simulink library "frdc"  (Simulink 8.1)
settings: Solver=ode1  StartTime=0.0  StopTime=Inf  FixedStep=0.001  RelTol=1e-3
PostLoadFcn:
  | , if any(exist('dsrtsu_mdlpostloadfcn', 'file') == [2, 3, 6]), try dsrtsu_mdlpostloadfcn('Execute', bdroot); catch fprintf('Error in PostLoadFcn (dsrtsu_mdlpostloadfcn) for model "%s":\n %s\n', bdroot, lasterr); end, end,
settings Model: DSRTSU_INTERNAL_RTI_VER=450  DSRTSU_INTERNAL_RTI_TYPE=rti1401  Creator=tescamilla  LastModifiedBy=tescamilla

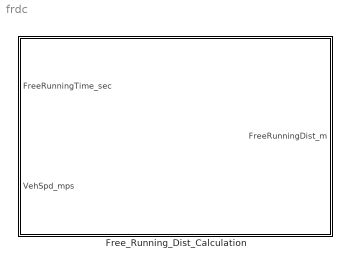
== system frdc ==
  Free_Running_Dist_Calculation : Subsystem

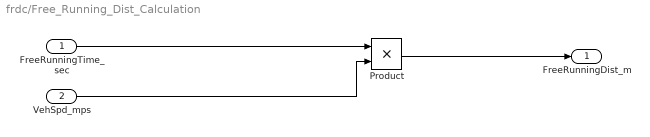
== system frdc/Free_Running_Dist_Calculation ==
  FreeRunningTime_sec : Inport
  VehSpd_mps : Inport  Port=2
  Product : Product
  FreeRunningDist_m : Outport
  wires:
  Product/1 -> FreeRunningDist_m/1
  VehSpd_mps/1 -> Product/2
  FreeRunningTime_sec/1 -> Product/1
